simulink model "G3P3_Demo"  (R2023a)
settings: Solver=FixedStepAuto  StartTime=0  StopTime=86400  FixedStep=10  RelTol=1e-3  EnableMultiTasking=on
settings Model: Creator=Owner  LastModifiedBy=Owner
settings SolverCC: AutoInsertRateTranBlk=on
settings HardwareCC: ProdBitPerLong=64  ProdHWDeviceType=Intel->x86-64 (Linux 64)
settings ModelReferenceCC: EnableRefExpFcnMdlSchedulingChecks=on  EnableParallelModelReferenceBuilds=on  ParallelModelReferenceMATLABWorkerInit=Load Top Model
settings RTWCC: Description=Simulink Desktop Real-Time  SystemTargetFile=sldrt.tlc  GenCodeOnly=on  TemplateMakefile=sldrt.tmf  TargetLang=C++  RTWCompilerOptimization=on
settings CodeAppCC: MaxIdLength=95
settings SimulinkDesktopRealTimeCC: TargetLibSuffix=_sldrt.a  TargetPreCompLibLocation=C:\Program Files\MATLAB\R2023a\toolbox\sldrt\lib\win64  TargetLangStandard=C++11 (ISO)

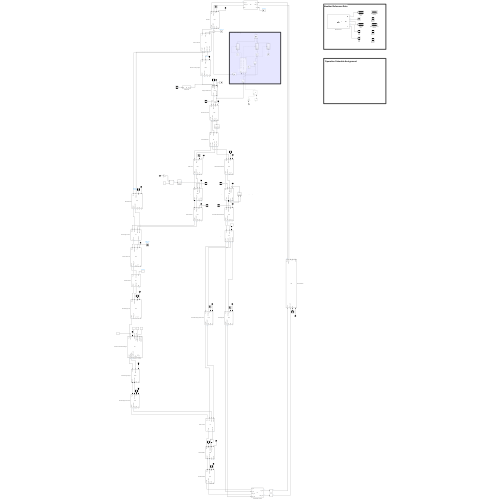
[thumbnail: Simulink's stored preview of the top-level diagram]
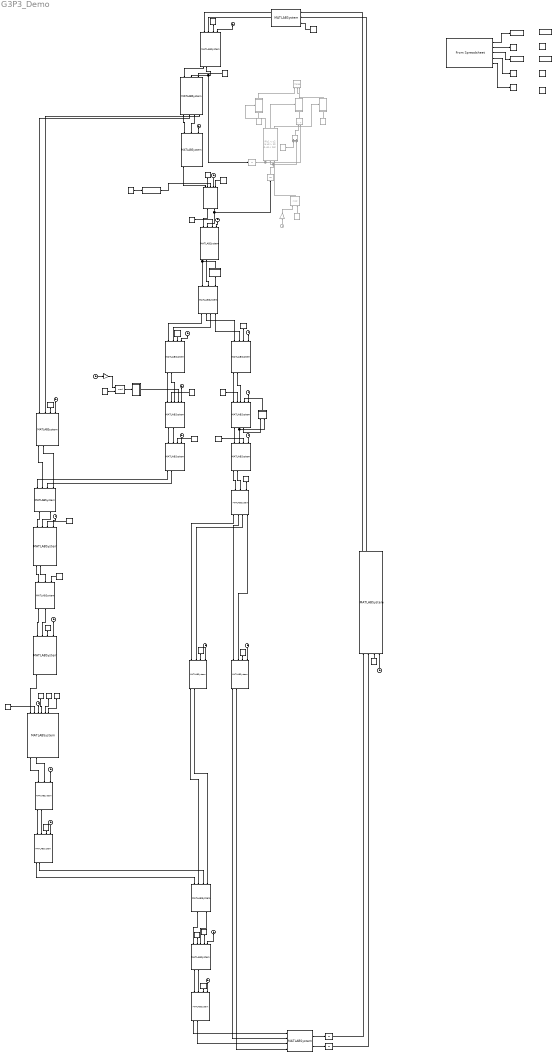
== system G3P3_Demo ==
  note: Operation Schedule Assignment
  note: Weather Reference Data
  note: Reciever Flow Rate Logic
  ABQ TMY3 Data : FromSpreadsheet  FileName=ABQ_Weather_Lookup.xlsx  OutDataTypeStr=double
  Add : Sum  Commented=on
  Bucket Elevator : MATLABSystem  System=BE  n=100  W=1  L=2  H=50  tm=0.006  SimulateUsing=Code generation  Ts0=20  Tm0=20  cp_s=1250  rho_s=3500  phi_s=0.6  cp_m=500  rho_m=8000  hinf=10  hsw=180
      mask Type: BE
      mask Display:
      | disp('BE');
      | port_label('input',1,'Ts_in');
      | port_label('input',2,'mdot_s_in');
      | port_label('input',3,'Tinf');
      | port_label('input',4,'t');
      | port_label('output',1,'Ts_out');
      | port_label('output',2,'mdot_s_out');
      | port_label('output',3,'Ts');
      | port_label('output',4,'Tm');
      | port_label('output',5,'x');
      | port_label('output',6,'qloss');
  Bucket Elevator Junction : MATLABSystem  System=SJ  cp_s=1250  Tref=0  SimulateUsing=Code generation
      mask Type: SJ
      mask Display:
      | disp('SJ');
      | port_label('input',1,'Ts_in1');
      | port_label('input',2,'Ts_in2');
      | port_label('input',3,'mdot_in1');
      | port_label('input',4,'mdot_in2');
      | port_label('output',1,'Ts_out');
      | port_label('output',2,'mdot_out');
  Clock{,1..21} (22 alike) : Clock
  Clock22 : Clock  Commented=on
  Cold Bin Bypass : MATLABSystem  System=FFD  n=100  D=0.25  L=1  td=0.003  SimulateUsing=Code generation  Ts0=25  Tm0=25  cp_s=1250  rho_s=3500  phi_s=0.6  cp_m=500  rho_m=8000  hinf=10  hsw=100
      mask Type: FFD
      mask Display:
      | disp('FFD');
      | port_label('input',1,'Ts_in');
      | port_label('input',2,'mdot_s_in');
      | port_label('input',3,'Tinf');
      | port_label('input',4,'t');
      | port_label('output',1,'Ts_out');
      | port_label('output',2,'mdot_s_out');
      | port_label('output',3,'Ts');
      | port_label('output',4,'Tm');
      | port_label('output',5,'x');
  Cold Bin Discharge : MATLABSystem  System=FFD  n=100  D=0.25  L=1  td=0.003  SimulateUsing=Code generation  Ts0=25  Tm0=25  cp_s=1250  rho_s=3500  phi_s=0.6  cp_m=500  rho_m=8000  hinf=10  hsw=100
      mask Type: FFD
      mask Display:
      | disp('FFD');
      | port_label('input',1,'Ts_in');
      | port_label('input',2,'mdot_s_in');
      | port_label('input',3,'Tinf');
      | port_label('input',4,'t');
      | port_label('output',1,'Ts_out');
      | port_label('output',2,'mdot_s_out');
      | port_label('output',3,'Ts');
      | port_label('output',4,'Tm');
      | port_label('output',5,'x');
  Cold Bin Junction : MATLABSystem  System=SJ  cp_s=1250  Tref=0  SimulateUsing=Code generation
      mask Type: SJ
      mask Display:
      | disp('SJ');
      | port_label('input',1,'Ts_in1');
      | port_label('input',2,'Ts_in2');
      | port_label('input',3,'mdot_in1');
      | port_label('input',4,'mdot_in2');
      | port_label('output',1,'Ts_out');
      | port_label('output',2,'mdot_out');
  Cold Storage Bin : MATLABSystem  System=LSB  H=7  D=5  SimulateUsing=Code generation  ms0=119000  Ts0=615  ht=0.25  hinf=10  cp_s=1250  rho_s=3500  phi_s=0.9
      mask Type: LSB
      mask Display:
      | disp('LSB');
      | port_label('input',1,'Ts_in');
      | port_label('input',2,'Tinf');
      | port_label('input',3,'mdot_s_in');
      | port_label('input',4,'mdot_s_out');
      | port_label('input',5,'t');
      | port_label('output',1,'Ts_out');
      | port_label('output',2,'mdot_s_out');
      | port_label('output',3,'ms');
      | port_label('output',4,'qloss');
  Cold Storage Diverter : MATLABSystem  System=SS  SimulateUsing=Code generation
      mask Type: SS
      mask Display:
      | disp('SS');
      | port_label('input',1,'Ts_in');
      | port_label('input',2,'mdot_in');
      | port_label('input',3,'y1');
      | port_label('output',1,'Ts_out1');
      | port_label('output',2,'Ts_out2');
      | port_label('output',3,'mdot_out1');
      | port_label('output',4,'mdot_out2');
  Constant : Constant  Value=775
  Constant1 : Constant  Commented=on
  Constant10 : Constant  Value=700
  Constant11 : Constant  Value=5
  Constant12 : Constant  Commented=on  Value=0
  Constant13 : Constant  Value=600
  Constant14 : Constant
  Constant2 : Constant
  Constant3 : Constant  Value=750
  Constant4 : Constant  Commented=on  Value=1e-6
  Constant5 : Constant  Commented=on  Value=24
  Constant6 : Constant  Value=0.5
  Constant7 : Constant  Value=24
  Constant8 : Constant  Value=565
  Constant9 : Constant  Value=601
  DNI Store Memory : DataStoreMemory  DataStoreName=DNI  WriteAfterWriteMsg=warning  ShowAdditionalParam=off
  DNI Uncertainty Store Memory : DataStoreMemory  DataStoreName=DNIuncert  WriteAfterWriteMsg=warning  ShowAdditionalParam=off
  DNI Write : DataStoreWrite  DataStoreName=DNI  IndexOptions=Index vector (dialog)  Indices=1  OutputSizes=1
  DNIuncert Write : DataStoreWrite  DataStoreName=DNIuncert  IndexOptions=Index vector (dialog)  Indices=1  OutputSizes=1
  Data Store Read : DataStoreRead  DataStoreName=DNI  IndexOptions=Index vector (dialog)  Indices=1  OutputSizes=1
  Data Store Read{1..18} (18 alike) : DataStoreRead  DataStoreName=Tinf  IndexOptions=Index vector (dialog)  Indices=1  OutputSizes=1
  Divide : Product  Commented=on  Inputs=*/
  Electric Heater Inlet : MATLABSystem  System=FFD  n=100  D=0.25  L=1  td=0.003  SimulateUsing=Code generation  Ts0=25  Tm0=25  cp_s=1250  rho_s=3500  phi_s=0.6  cp_m=500  rho_m=8000  hinf=10  hsw=100
      mask Type: FFD
      mask Display:
      | disp('FFD');
      | port_label('input',1,'Ts_in');
      | port_label('input',2,'mdot_s_in');
      | port_label('input',3,'Tinf');
      | port_label('input',4,'t');
      | port_label('output',1,'Ts_out');
      | port_label('output',2,'mdot_s_out');
      | port_label('output',3,'Ts');
      | port_label('output',4,'Tm');
      | port_label('output',5,'x');
  FPR Inlet : MATLABSystem  System=FFD  n=100  D=0.25  L=1  td=0.003  SimulateUsing=Code generation  Ts0=25  Tm0=25  cp_s=1250  rho_s=3500  phi_s=0.6  cp_m=500  rho_m=8000  hinf=10  hsw=100
      mask Type: FFD
      mask Display:
      | disp('FFD');
      | port_label('input',1,'Ts_in');
      | port_label('input',2,'mdot_s_in');
      | port_label('input',3,'Tinf');
      | port_label('input',4,'t');
      | port_label('output',1,'Ts_out');
      | port_label('output',2,'mdot_s_out');
      | port_label('output',3,'Ts');
      | port_label('output',4,'Tm');
      | port_label('output',5,'x');
  Falling Particle Receiver : MATLABSystem  System=FPR  H=1.2  W=1.2  d=0.0417  SimulateUsing=Code generation  Ts0=600  hInf=5  cp_s=1250  rho_s=3500  phi_s=0.6  epsilon_s=0.88  alpha_s=0.92  tauLag=500  tauLead=100
      mask Type: FPR
      mask Display:
      | disp('FPR');
      | port_label('input',1,'Ts_in');
      | port_label('input',2,'Tinf');
      | port_label('input',3,'Qsolar');
      | port_label('input',4,'t');
      | port_label('input',5,'Tset');
      | port_label('output',1,'Ts_out');
      | port_label('output',2,'mdot_s_out');
  Gain : Gain  Gain=1/3600
  Gain1 : Gain  Commented=on  Gain=1/3600
  HX Electric Heater : MATLABSystem  System=EH  cp_s=1250  SimulateUsing=Code generation
      mask Type: EH
      mask Display:
      | disp('EH');
      | port_label('input',1,'Ts_in');
      | port_label('input',2,'mdot_in');
      | port_label('input',3,'Tset');
      | port_label('output',1,'Ts_out');
      | port_label('output',2,'mdot_out');
      | port_label('output',3,'Qin');
  Heat Exchanger Down Comer : MATLABSystem  System=FFD  n=100  D=0.25  L=1  td=0.003  SimulateUsing=Code generation  Ts0=25  Tm0=25  cp_s=1250  rho_s=3500  phi_s=0.6  cp_m=500  rho_m=8000  hinf=10  hsw=100
      mask Type: FFD
      mask Display:
      | disp('FFD');
      | port_label('input',1,'Ts_in');
      | port_label('input',2,'mdot_s_in');
      | port_label('input',3,'Tinf');
      | port_label('input',4,'t');
      | port_label('output',1,'Ts_out');
      | port_label('output',2,'mdot_s_out');
      | port_label('output',3,'Ts');
      | port_label('output',4,'Tm');
      | port_label('output',5,'x');
  Heat Exchanger Hopper : MATLABSystem  System=MFH  n=20  H=1  D=1.2  SimulateUsing=Code generation  Ts0=25  cp_s=1250  rho_s=3500  phi_s=0.6
      mask Type: MFH
      mask Display:
      | disp('MFH');
      | port_label('input',1,'Ts_in');
      | port_label('input',2,'mdot_s_in');
      | port_label('input',3,'t');
      | port_label('output',1,'Ts_out');
      | port_label('output',2,'mdot_s_out');
      | port_label('output',3,'Ts');
      | port_label('output',4,'x');
  Heat Exchanger Inlet : MATLABSystem  System=FFD  n=100  D=0.25  L=1  td=0.003  SimulateUsing=Code generation  Ts0=25  Tm0=25  cp_s=1250  rho_s=3500  phi_s=0.6  cp_m=500  rho_m=8000  hinf=10  hsw=100
      mask Type: FFD
      mask Display:
      | disp('FFD');
      | port_label('input',1,'Ts_in');
      | port_label('input',2,'mdot_s_in');
      | port_label('input',3,'Tinf');
      | port_label('input',4,'t');
      | port_label('output',1,'Ts_out');
      | port_label('output',2,'mdot_s_out');
      | port_label('output',3,'Ts');
      | port_label('output',4,'Tm');
      | port_label('output',5,'x');
  Heat Exchanger Junction : MATLABSystem  System=SJ  cp_s=1250  Tref=0  SimulateUsing=Code generation
      mask Type: SJ
      mask Display:
      | disp('SJ');
      | port_label('input',1,'Ts_in1');
      | port_label('input',2,'Ts_in2');
      | port_label('input',3,'mdot_in1');
      | port_label('input',4,'mdot_in2');
      | port_label('output',1,'Ts_out');
      | port_label('output',2,'mdot_out');
  Heliostat Field : MATLABSystem  System=HF  n=150  H=5  W=5  eta_op=0.6  SimulateUsing=Code generation
      mask Type: HF
      mask Display:
      | disp('HF');
      | port_label('input',1,'DNI');
      | port_label('output',1,'Q_rec');
  Hot Bin Discharge : MATLABSystem  System=FFD  n=100  D=0.25  L=1  td=0.003  SimulateUsing=Code generation  Ts0=25  Tm0=25  cp_s=1250  rho_s=3500  phi_s=0.6  cp_m=500  rho_m=8000  hinf=10  hsw=100
      mask Type: FFD
      mask Display:
      | disp('FFD');
      | port_label('input',1,'Ts_in');
      | port_label('input',2,'mdot_s_in');
      | port_label('input',3,'Tinf');
      | port_label('input',4,'t');
      | port_label('output',1,'Ts_out');
      | port_label('output',2,'mdot_s_out');
      | port_label('output',3,'Ts');
      | port_label('output',4,'Tm');
      | port_label('output',5,'x');
  Hot Bin Inlet : MATLABSystem  System=FFD  n=100  D=0.25  L=10  td=0.003  SimulateUsing=Code generation  Ts0=25  Tm0=25  cp_s=1250  rho_s=3500  phi_s=0.6  cp_m=500  rho_m=8000  hinf=10  hsw=100
      mask Type: FFD
      mask Display:
      | disp('FFD');
      | port_label('input',1,'Ts_in');
      | port_label('input',2,'mdot_s_in');
      | port_label('input',3,'Tinf');
      | port_label('input',4,'t');
      | port_label('output',1,'Ts_out');
      | port_label('output',2,'mdot_s_out');
      | port_label('output',3,'Ts');
      | port_label('output',4,'Tm');
      | port_label('output',5,'x');
  Hot Storage Bin : MATLABSystem  System=LSB  H=7  D=5  SimulateUsing=Code generation  ms0=232492  Ts0=775  ht=0.25  hinf=10  cp_s=1250  rho_s=3500  phi_s=0.9
      mask Type: LSB
      mask Display:
      | disp('LSB');
      | port_label('input',1,'Ts_in');
      | port_label('input',2,'Tinf');
      | port_label('input',3,'mdot_s_in');
      | port_label('input',4,'mdot_s_out');
      | port_label('input',5,'t');
      | port_label('output',1,'Ts_out');
      | port_label('output',2,'mdot_s_out');
      | port_label('output',3,'ms');
      | port_label('output',4,'qloss');
  Hot Storage Discharge Logic : Subsystem
  Hot Storage Diverter : MATLABSystem  System=SS  SimulateUsing=Code generation
      mask Type: SS
      mask Display:
      | disp('SS');
      | port_label('input',1,'Ts_in');
      | port_label('input',2,'mdot_in');
      | port_label('input',3,'y1');
      | port_label('output',1,'Ts_out1');
      | port_label('output',2,'Ts_out2');
      | port_label('output',3,'mdot_out1');
      | port_label('output',4,'mdot_out2');
  If : If  Commented=on  NumInputs=3  IfExpression=u1 < u2 & u3 > 10 & u3 < 16  ElseIfExpressions=u1 > u2 & u3 > 10 & u3 < 16
  If Action Subsystem : Subsystem  Commented=on  TreatAsAtomicUnit=on
  If Action Subsystem1 : Subsystem  Commented=on  TreatAsAtomicUnit=on
  If Action Subsystem2 : Subsystem  Commented=on  TreatAsAtomicUnit=on
  Intermediate Storage Bin : MATLABSystem  System=LSB  H=6  D=1.13  SimulateUsing=Code generation  ms0=1  Ts0=615  ht=0.25  hinf=10  cp_s=1250  rho_s=3500  phi_s=0.98
      mask Type: LSB
      mask Display:
      | disp('LSB');
      | port_label('input',1,'Ts_in');
      | port_label('input',2,'Tinf');
      | port_label('input',3,'mdot_s_in');
      | port_label('input',4,'mdot_s_out');
      | port_label('input',5,'t');
      | port_label('output',1,'Ts_out');
      | port_label('output',2,'mdot_s_out');
      | port_label('output',3,'ms');
      | port_label('output',4,'qloss');
  Intermediate Storage Bin Logic : Subsystem
  Intermediate Storage Discharge : MATLABSystem  System=FFD  n=100  D=0.25  L=1  td=0.003  SimulateUsing=Code generation  Ts0=25  Tm0=25  cp_s=1250  rho_s=3500  phi_s=0.6  cp_m=500  rho_m=8000  hinf=10  hsw=100
      mask Type: FFD
      mask Display:
      | disp('FFD');
      | port_label('input',1,'Ts_in');
      | port_label('input',2,'mdot_s_in');
      | port_label('input',3,'Tinf');
      | port_label('input',4,'t');
      | port_label('output',1,'Ts_out');
      | port_label('output',2,'mdot_s_out');
      | port_label('output',3,'Ts');
      | port_label('output',4,'Tm');
      | port_label('output',5,'x');
  Intermediate Storage Down Comer : MATLABSystem  System=FFD  n=100  D=0.25  L=1  td=0.003  SimulateUsing=Code generation  Ts0=25  Tm0=25  cp_s=1250  rho_s=3500  phi_s=0.6  cp_m=500  rho_m=8000  hinf=10  hsw=100
      mask Type: FFD
      mask Display:
      | disp('FFD');
      | port_label('input',1,'Ts_in');
      | port_label('input',2,'mdot_s_in');
      | port_label('input',3,'Tinf');
      | port_label('input',4,'t');
      | port_label('output',1,'Ts_out');
      | port_label('output',2,'mdot_s_out');
      | port_label('output',3,'Ts');
      | port_label('output',4,'Tm');
      | port_label('output',5,'x');
  Intermediate Storage Inlet : MATLABSystem  System=FFD  n=100  D=0.25  L=10  td=0.003  SimulateUsing=Code generation  Ts0=25  Tm0=25  cp_s=1250  rho_s=3500  phi_s=0.6  cp_m=500  rho_m=8000  hinf=10  hsw=100
      mask Type: FFD
      mask Display:
      | disp('FFD');
      | port_label('input',1,'Ts_in');
      | port_label('input',2,'mdot_s_in');
      | port_label('input',3,'Tinf');
      | port_label('input',4,'t');
      | port_label('output',1,'Ts_out');
      | port_label('output',2,'mdot_s_out');
      | port_label('output',3,'Ts');
      | port_label('output',4,'Tm');
      | port_label('output',5,'x');
  MATLAB System : MATLABSystem  System=EH  cp_s=1250  SimulateUsing=Code generation
      mask Type: EH
      mask Display:
      | disp('EH');
      | port_label('input',1,'Ts_in');
      | port_label('input',2,'mdot_in');
      | port_label('input',3,'Tset');
      | port_label('output',1,'Ts_out');
      | port_label('output',2,'mdot_out');
      | port_label('output',3,'Qin');
  Merge : Merge  Commented=on  Inputs=3
  Mod : Math  Operator=mod
  Mod1 : Math  Commented=on  Operator=mod
  Particle-to-sCO2 Heat Exchanger : MATLABSystem  System=HX  n=20  t_s=0.006  t_CO2=0.001  t_m=0.003  H=1.5  W=0.6  N_plate=33  SimulateUsing=Code generation  Ts0=600  Tco20=600  Tm0=25  h_s=450  h_CO2=3000  cp_s=1250  rho_s=3500  phi_s=0.6  cp_CO2=1250  rho_CO2=110  cp_m=500  rho_m=8000
      mask Type: HX
      mask Display:
      | disp('HX');
      | port_label('input',1,'Ts_in');
      | port_label('input',2,'Tco2_in');
      | port_label('input',3,'t');
      | port_label('input',4,'mode');
      | port_label('input',5,'Ts_out_set');
      | port_label('input',6,'Tco2_out_set');
      | port_label('input',7,'mdot_s_in');
      | port_label('input',8,'mdot_CO2_in');
      | port_label('output',1,'Ts_out');
      | port_label('output',2,'Tco2_out');
      | port_label('output',3,'mdot_s_out');
      | port_label('output',4,'mdot_CO2_out');
      | port_label('output',5,'Ts');
      | port_label('output',6,'Tco2');
      | port_label('output',7,'Tm');
      | port_label('output',8,'Q_CO2');
      | port_label('output',9,'Q_s');
      | port_label('output',10,'x');
  Receiver Bypass : MATLABSystem  System=FFD  n=100  D=0.25  L=1  td=0.003  SimulateUsing=Code generation  Ts0=25  Tm0=25  cp_s=1250  rho_s=3500  phi_s=0.6  cp_m=500  rho_m=8000  hinf=10  hsw=100
      mask Type: FFD
      mask Display:
      | disp('FFD');
      | port_label('input',1,'Ts_in');
      | port_label('input',2,'mdot_s_in');
      | port_label('input',3,'Tinf');
      | port_label('input',4,'t');
      | port_label('output',1,'Ts_out');
      | port_label('output',2,'mdot_s_out');
      | port_label('output',3,'Ts');
      | port_label('output',4,'Tm');
      | port_label('output',5,'x');
  Receiver Diverter : MATLABSystem  System=SS  SimulateUsing=Code generation
      mask Type: SS
      mask Display:
      | disp('SS');
      | port_label('input',1,'Ts_in');
      | port_label('input',2,'mdot_in');
      | port_label('input',3,'y1');
      | port_label('output',1,'Ts_out1');
      | port_label('output',2,'Ts_out2');
      | port_label('output',3,'mdot_out1');
      | port_label('output',4,'mdot_out2');
  Receiver Down Comer : MATLABSystem  System=FFD  n=100  D=0.25  L=10  td=0.003  SimulateUsing=Code generation  Ts0=25  Tm0=25  cp_s=1250  rho_s=3500  phi_s=0.6  cp_m=500  rho_m=8000  hinf=10  hsw=100
      mask Type: FFD
      mask Display:
      | disp('FFD');
      | port_label('input',1,'Ts_in');
      | port_label('input',2,'mdot_s_in');
      | port_label('input',3,'Tinf');
      | port_label('input',4,'t');
      | port_label('output',1,'Ts_out');
      | port_label('output',2,'mdot_s_out');
      | port_label('output',3,'Ts');
      | port_label('output',4,'Tm');
      | port_label('output',5,'x');
  Receiver Inventory Hopper : MATLABSystem  System=MFH  n=20  H=1  D=1.2  SimulateUsing=Code generation  Ts0=25  cp_s=1250  rho_s=3500  phi_s=0.6
      mask Type: MFH
      mask Display:
      | disp('MFH');
      | port_label('input',1,'Ts_in');
      | port_label('input',2,'mdot_s_in');
      | port_label('input',3,'t');
      | port_label('output',1,'Ts_out');
      | port_label('output',2,'mdot_s_out');
      | port_label('output',3,'Ts');
      | port_label('output',4,'x');
  Storage Diverter Logic : Subsystem
  TMY3 Hour Store Memory : DataStoreMemory  DataStoreName=TMY3hour  WriteAfterWriteMsg=warning  ShowAdditionalParam=off
  TMY3hour Write : DataStoreWrite  DataStoreName=TMY3hour  IndexOptions=Index vector (dialog)  Indices=1  OutputSizes=1
  Tinf Write : DataStoreWrite  DataStoreName=Tinf  IndexOptions=Index vector (dialog)  Indices=1  OutputSizes=1
  Tinf Store Memory : DataStoreMemory  DataStoreName=Tinf  WriteAfterWriteMsg=warning  ShowAdditionalParam=off
  Uinf Write : DataStoreWrite  DataStoreName=Uinf  IndexOptions=Index vector (dialog)  Indices=1  OutputSizes=1
  Uinf Store Memory : DataStoreMemory  DataStoreName=Uinf  WriteAfterWriteMsg=warning  ShowAdditionalParam=off
  Unit Delay : UnitDelay  InitialCondition=600  SampleTime=-1  HasFrameUpgradeWarning=on
  Unit Delay1 : UnitDelay  InitialCondition=1e-5  SampleTime=-1  HasFrameUpgradeWarning=on
  Unit Delay2 : UnitDelay  Commented=on  SampleTime=-1  HasFrameUpgradeWarning=on
  Unit Delay3 : UnitDelay  Commented=on  SampleTime=-1  HasFrameUpgradeWarning=on
  wires:
  Clock1/1 -> Falling Particle Receiver/4
  Heliostat Field/1 -> Falling Particle Receiver/3
  Constant/1 -> Falling Particle Receiver/5
  Falling Particle Receiver/1 -> Receiver Down Comer/1
  Clock2/1 -> Receiver Down Comer/4
  Receiver Down Comer/1 -> Storage Diverter Logic/1(In1), Hot Storage Diverter/1
  Receiver Down Comer/2 -> Hot Storage Diverter/2
  Storage Diverter Logic/1(Out1) -> Hot Storage Diverter/3
  Hot Storage Diverter/1 -> Hot Bin Inlet/1
  Hot Storage Diverter/3 -> Hot Bin Inlet/2
  Clock3/1 -> Hot Bin Inlet/4
  Hot Storage Diverter/2 -> Intermediate Storage Inlet/1
  Hot Storage Diverter/4 -> Intermediate Storage Inlet/2
  Hot Bin Inlet/1 -> Hot Storage Bin/1
  Hot Bin Inlet/2 -> Hot Storage Bin/3
  Clock4/1 -> Hot Storage Bin/5
  Intermediate Storage Inlet/1 -> Intermediate Storage Bin/1
  Intermediate Storage Inlet/2 -> Intermediate Storage Bin/3
  Hot Storage Bin/1 -> Hot Bin Discharge/1
  Hot Storage Bin/2 -> Hot Bin Discharge/2
  Clock5/1 -> Hot Bin Discharge/4
  Clock6/1 -> Intermediate Storage Bin/5
  Clock7/1 -> Intermediate Storage Discharge/4
  Intermediate Storage Bin/1 -> Intermediate Storage Discharge/1
  Intermediate Storage Bin/2 -> Intermediate Storage Discharge/2, Intermediate Storage Bin Logic/2(In2)
  Hot Bin Discharge/1 -> Heat Exchanger Junction/1
  Hot Bin Discharge/2 -> Heat Exchanger Junction/3
  Intermediate Storage Discharge/1 -> Cold Storage Diverter/1
  Intermediate Storage Discharge/2 -> Cold Storage Diverter/2
  Constant6/1 -> Cold Storage Diverter/3
  Clock/1 -> Gain/1
  Gain/1 -> Mod/1
  Constant7/1 -> Mod/2
  Mod/1 -> Hot Storage Discharge Logic/1(In1)
  Hot Storage Discharge Logic/1(Out1) -> Hot Storage Bin/4
  Clock8/1 -> Intermediate Storage Inlet/4
  Intermediate Storage Bin/3 -> Intermediate Storage Bin Logic/1(In1)
  Intermediate Storage Bin Logic/1(Out1) -> Intermediate Storage Bin/4
  Clock9/1 -> Particle-to-sCO2 Heat Exchanger/3
  Constant2/1 -> Particle-to-sCO2 Heat Exchanger/4
  Constant3/1 -> HX Electric Heater/3
  Constant8/1 -> Particle-to-sCO2 Heat Exchanger/2
  Constant9/1 -> Particle-to-sCO2 Heat Exchanger/5
  Constant10/1 -> Particle-to-sCO2 Heat Exchanger/6
  Particle-to-sCO2 Heat Exchanger/1 -> Heat Exchanger Hopper/1
  Particle-to-sCO2 Heat Exchanger/3 -> Heat Exchanger Hopper/2
  Clock10/1 -> Heat Exchanger Hopper/3
  Heat Exchanger Hopper/1 -> Heat Exchanger Down Comer/1
  Heat Exchanger Hopper/2 -> Heat Exchanger Down Comer/2
  Heat Exchanger Junction/1 -> Electric Heater Inlet/1
  Heat Exchanger Junction/2 -> Electric Heater Inlet/2
  Clock11/1 -> Electric Heater Inlet/4
  Electric Heater Inlet/1 -> HX Electric Heater/1
  Electric Heater Inlet/2 -> HX Electric Heater/2
  HX Electric Heater/1 -> Heat Exchanger Inlet/1
  HX Electric Heater/2 -> Heat Exchanger Inlet/2
  Clock12/1 -> Heat Exchanger Inlet/4
  Heat Exchanger Inlet/1 -> Particle-to-sCO2 Heat Exchanger/1
  Clock13/1 -> Heat Exchanger Down Comer/4
  Heat Exchanger Down Comer/2 -> Cold Bin Junction/3
  Heat Exchanger Down Comer/1 -> Cold Bin Junction/1
  Cold Storage Diverter/1 -> Intermediate Storage Down Comer/1
  Cold Storage Diverter/3 -> Intermediate Storage Down Comer/2
  Clock14/1 -> Intermediate Storage Down Comer/4
  Intermediate Storage Down Comer/1 -> Cold Bin Junction/2
  Intermediate Storage Down Comer/2 -> Cold Bin Junction/4
  Cold Storage Diverter/2 -> Cold Bin Bypass/1
  Cold Storage Diverter/4 -> Cold Bin Bypass/2
  Clock15/1 -> Cold Bin Bypass/4
  Cold Bin Junction/1 -> Cold Storage Bin/1
  Cold Bin Junction/2 -> Cold Storage Bin/3
  Clock16/1 -> Cold Storage Bin/5
  Constant11/1 -> Cold Storage Bin/4
  Cold Storage Bin/1 -> Cold Bin Discharge/1
  Cold Storage Bin/2 -> Cold Bin Discharge/2
  Clock17/1 -> Cold Bin Discharge/4
  Cold Bin Discharge/1 -> Bucket Elevator Junction/1
  Cold Bin Discharge/2 -> Bucket Elevator Junction/3
  Cold Bin Bypass/1 -> Bucket Elevator Junction/2
  Cold Bin Bypass/2 -> Bucket Elevator Junction/4
  Unit Delay/1 -> Bucket Elevator/1
  Unit Delay1/1 -> Bucket Elevator/2
  Clock18/1 -> Bucket Elevator/4
  FPR Inlet/1 -> Receiver Diverter/1
  Receiver Diverter/1 -> Receiver Inventory Hopper/1
  Receiver Diverter/3 -> Receiver Inventory Hopper/2
  Clock19/1 -> Receiver Inventory Hopper/3
  Receiver Inventory Hopper/1 -> Falling Particle Receiver/1
  Bucket Elevator/1 -> MATLAB System/1
  Bucket Elevator/2 -> MATLAB System/2
  Clock20/1 -> FPR Inlet/4
  Bucket Elevator Junction/1 -> Unit Delay/1
  Bucket Elevator Junction/2 -> Unit Delay1/1
  Clock21/1 -> Receiver Bypass/4
  Receiver Diverter/2 -> Receiver Bypass/1
  Receiver Diverter/4 -> Receiver Bypass/2
  Receiver Bypass/1 -> Heat Exchanger Junction/2
  Receiver Bypass/2 -> Heat Exchanger Junction/4
  Add/1 -> Divide/1
  Constant4/1 -> Add/1
  If/1 -> If Action Subsystem/Action
  If Action Subsystem1/1(Out1) -> Merge/2
  Divide/1 -> If Action Subsystem1/1(In1)
  FPR Inlet/2 -> Unit Delay3/1, Receiver Diverter/2
  If Action Subsystem/1(Out1) -> Merge/1
  Falling Particle Receiver/2 -> Unit Delay2/1, Receiver Down Comer/2
  Unit Delay2/1 -> If/2, Add/2
  Constant1/1 -> If Action Subsystem/1(In1)
  Clock22/1 -> Gain1/1
  Constant5/1 -> Mod1/2
  Gain1/1 -> Mod1/1
  Mod1/1 -> If/3
  If/2 -> If Action Subsystem1/Action
  If/3 -> If Action Subsystem2/Action
  Constant12/1 -> If Action Subsystem2/1(In1)
  If Action Subsystem2/1(Out1) -> Merge/3
  ABQ TMY3 Data/2 -> DNI Write/1
  Data Store Read/1 -> Heliostat Field/1
  ABQ TMY3 Data/3 -> DNIuncert Write/1
  ABQ TMY3 Data/4 -> Tinf Write/1
  ABQ TMY3 Data/5 -> Uinf Write/1
  ABQ TMY3 Data/1 -> TMY3hour Write/1
  Data Store Read1/1 -> FPR Inlet/3
  Data Store Read2/1 -> Falling Particle Receiver/2
  Data Store Read3/1 -> Receiver Down Comer/3
  Data Store Read4/1 -> Hot Bin Inlet/3
  Data Store Read5/1 -> Intermediate Storage Inlet/3
  Data Store Read6/1 -> Hot Storage Bin/2
  Data Store Read7/1 -> Intermediate Storage Bin/2
  Data Store Read8/1 -> Hot Bin Discharge/3
  Data Store Read9/1 -> Intermediate Storage Discharge/3
  Data Store Read10/1 -> Receiver Bypass/3
  Data Store Read11/1 -> Electric Heater Inlet/3
  Data Store Read12/1 -> Heat Exchanger Inlet/3
  Data Store Read13/1 -> Heat Exchanger Down Comer/3
  Data Store Read14/1 -> Intermediate Storage Down Comer/3
  Data Store Read15/1 -> Cold Bin Bypass/3
  Data Store Read16/1 -> Cold Storage Bin/2
  Data Store Read17/1 -> Cold Bin Discharge/3
  Data Store Read18/1 -> Bucket Elevator/3
  Constant13/1 -> MATLAB System/3
  MATLAB System/1 -> FPR Inlet/1
  MATLAB System/2 -> FPR Inlet/2
  Unit Delay3/1 -> Divide/2, If/1
  Constant14/1 -> Receiver Diverter/3

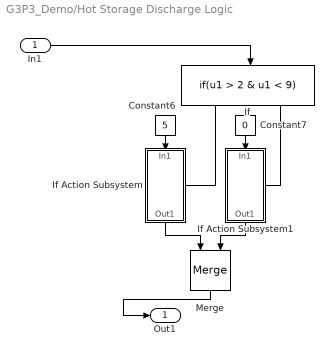
== system G3P3_Demo/Hot Storage Discharge Logic ==
  In1 : Inport
  Constant6 : Constant  Value=5
  Constant7 : Constant  Value=0
  If : If  IfExpression=u1 > 2 & u1 < 9
  If Action Subsystem : Subsystem  TreatAsAtomicUnit=on
  If Action Subsystem1 : Subsystem  TreatAsAtomicUnit=on
  Merge : Merge
  Out1 : Outport
  wires:
  If Action Subsystem1/1(Out1) -> Merge/2
  In1/1 -> If/1
  Constant6/1 -> If Action Subsystem/1(In1)
  Merge/1 -> Out1/1
  If Action Subsystem/1(Out1) -> Merge/1
  Constant7/1 -> If Action Subsystem1/1(In1)
  If/2 -> If Action Subsystem1/Action
  If/1 -> If Action Subsystem/Action

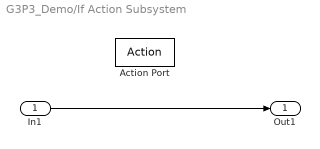
== system G3P3_Demo/If Action Subsystem ==
  In1 : Inport
  Action Port : ActionPort  ActionPortLabel=if(u1 < u2 & u3 > 10 & u3 < 16)
  Out1 : Outport
  wires:
  In1/1 -> Out1/1

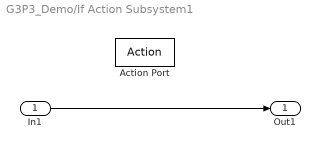
== system G3P3_Demo/If Action Subsystem1 ==
  In1 : Inport
  Action Port : ActionPort  ActionPortLabel=elseif(u1 > u2 & u3 > 10 & u3 < 16)
  Out1 : Outport
  wires:
  In1/1 -> Out1/1

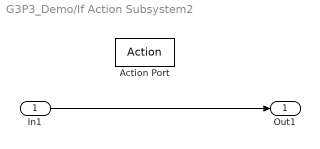
== system G3P3_Demo/If Action Subsystem2 ==
  In1 : Inport
  Action Port : ActionPort  ActionPortLabel=else
  Out1 : Outport
  wires:
  In1/1 -> Out1/1

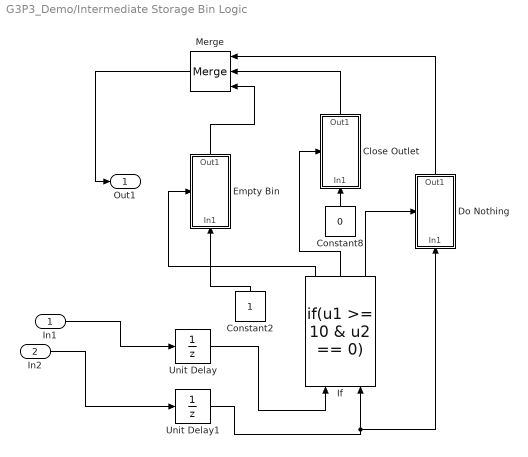
== system G3P3_Demo/Intermediate Storage Bin Logic ==
  In1 : Inport
  In2 : Inport  Port=2
  Close Outlet : Subsystem  TreatAsAtomicUnit=on
  Constant2 : Constant
  Constant8 : Constant  Value=0
  Do Nothing : Subsystem  TreatAsAtomicUnit=on
  Empty Bin : Subsystem  TreatAsAtomicUnit=on
  If : If  NumInputs=2  IfExpression=u1 >= 10 & u2 == 0  ElseIfExpressions=u1 <= 1 & u2 > 0
  Merge : Merge  Inputs=3
  Unit Delay : UnitDelay  SampleTime=-1  HasFrameUpgradeWarning=on
  Unit Delay1 : UnitDelay  SampleTime=-1  HasFrameUpgradeWarning=on
  Out1 : Outport
  wires:
  If/2 -> Close Outlet/Action
  Do Nothing/1(Out1) -> Merge/1
  Unit Delay/1 -> If/1
  Empty Bin/1(Out1) -> Merge/3
  In2/1 -> Unit Delay1/1
  Unit Delay1/1 -> Do Nothing/1(In1), If/2
  If/3 -> Do Nothing/Action
  In1/1 -> Unit Delay/1
  If/1 -> Empty Bin/Action
  Constant2/1 -> Empty Bin/1(In1)
  Constant8/1 -> Close Outlet/1(In1)
  Close Outlet/1(Out1) -> Merge/2
  Merge/1 -> Out1/1

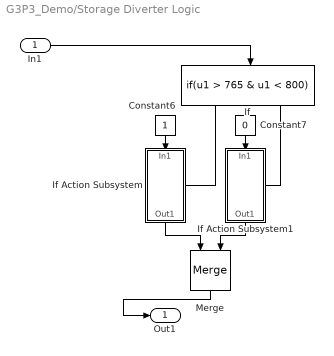
== system G3P3_Demo/Storage Diverter Logic ==
  In1 : Inport
  Constant6 : Constant
  Constant7 : Constant  Value=0
  If : If  IfExpression=u1 > 765 & u1 < 800
  If Action Subsystem : Subsystem  TreatAsAtomicUnit=on
  If Action Subsystem1 : Subsystem  TreatAsAtomicUnit=on
  Merge : Merge
  Out1 : Outport
  wires:
  If Action Subsystem1/1(Out1) -> Merge/2
  In1/1 -> If/1
  Constant6/1 -> If Action Subsystem/1(In1)
  Merge/1 -> Out1/1
  If Action Subsystem/1(Out1) -> Merge/1
  Constant7/1 -> If Action Subsystem1/1(In1)
  If/2 -> If Action Subsystem1/Action
  If/1 -> If Action Subsystem/Action

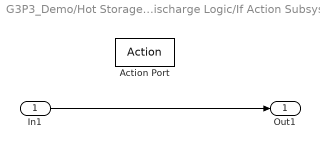
== system G3P3_Demo/Hot Storage Discharge Logic/If Action Subsystem ==
  In1 : Inport
  Action Port : ActionPort  ActionPortLabel=if(u1 > 2 & u1 < 9)
  Out1 : Outport
  wires:
  In1/1 -> Out1/1

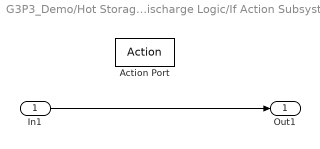
== system G3P3_Demo/Hot Storage Discharge Logic/If Action Subsystem1 ==
  In1 : Inport
  Action Port : ActionPort  ActionPortLabel=else
  Out1 : Outport
  wires:
  In1/1 -> Out1/1

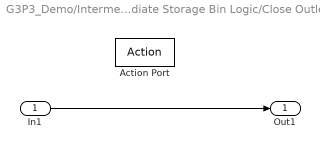
== system G3P3_Demo/Intermediate Storage Bin Logic/Close Outlet ==
  In1 : Inport
  Action Port : ActionPort  ActionPortLabel=elseif(u1 <= 1 & u2 > 0)
  Out1 : Outport
  wires:
  In1/1 -> Out1/1

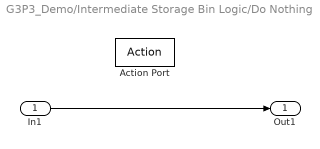
== system G3P3_Demo/Intermediate Storage Bin Logic/Do Nothing ==
  In1 : Inport
  Action Port : ActionPort  ActionPortLabel=else
  Out1 : Outport
  wires:
  In1/1 -> Out1/1

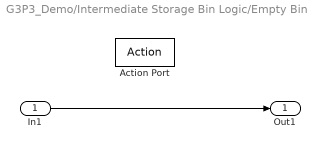
== system G3P3_Demo/Intermediate Storage Bin Logic/Empty Bin ==
  In1 : Inport
  Action Port : ActionPort  ActionPortLabel=if(u1 >= 10 & u2 == 0)
  Out1 : Outport
  wires:
  In1/1 -> Out1/1

== system G3P3_Demo/Storage Diverter Logic/If Action Subsystem ==
  In1 : Inport
  Action Port : ActionPort  ActionPortLabel=if(u1 > 765 & u1 < 800)
  Out1 : Outport
  wires:
  In1/1 -> Out1/1

== system G3P3_Demo/Storage Diverter Logic/If Action Subsystem1 ==
  In1 : Inport
  Action Port : ActionPort  ActionPortLabel=else
  Out1 : Outport
  wires:
  In1/1 -> Out1/1
